simulink model "modelOfSegway"  (R2016a)
settings: Solver=ode45  StartTime=0.0  StopTime=10  RelTol=1e-3
InitFcn:
  | start
  | control
values from neighbouring files (symbols this model uses):
  A = [0 0 1 ... (first row only)    [start.m]
  B = [0 ... (first row only)    [start.m]
  C = eye(3)    [start.m]
  D = 0.07    [params.m]    (also in start.m = zeros(3, 1))
  K = lqr(s1, QQ, RR)    [control.m]    (also in controlEV3.m = lqrd(s1.A,s1.B, QQ, RR, Ts); control_A.m = QQ*Inv(Y)*; control_P.m = (inv(AA)*BB)')
  K_PWM = 8.087    [params.m]
  Psi0 = 0.15    [params.m]
  R = 0.0275    [params.m]
  W = 0.08    [params.m]
libraries: simulink_extras x2
settings Model: Creator=Влад  LastModifiedBy=Влад
settings SolverCC: ZeroCrossAlgorithm=Adaptive

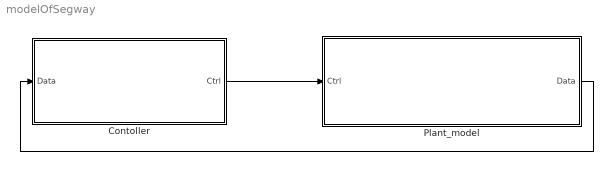
== system modelOfSegway ==
  Contoller : Subsystem
  Plant_model : Subsystem
  wires:
  Contoller/1(Ctrl) -> Plant_model/1(Ctrl)
  Plant_model/1(Data) -> Contoller/1(Data)

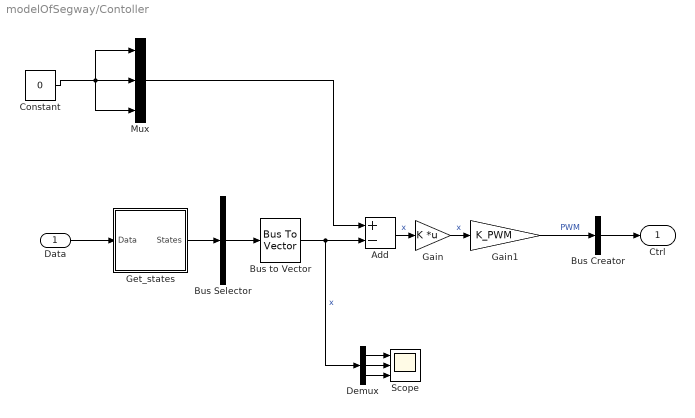
== system modelOfSegway/Contoller ==
  Data : Inport
  Add : Sum  Inputs=+-
  Bus Creator : BusCreator  Inputs=1  OutDataTypeStr=Bus: Ctrl
  Bus Selector : BusSelector  OutputSignals=psi,theta_dot,psi_dot  OutputAsBus=on
  Bus to Vector : BusToVector
  Constant : Constant  Value=0
  Demux : Demux  Outputs=3
  Gain : Gain  Gain=K  Multiplication=Matrix(K*u)
  Gain1 : Gain  Gain=K_PWM
  Get_states : Subsystem
  Mux : Mux  Inputs=3
  Scope : Scope  NumInputPorts=3
  Ctrl : Outport
  wires:
  Bus Creator/1 -> Ctrl/1
  Data/1 -> Get_states/1(Data)
  Get_states/1(States) -> Bus Selector/1
  Bus Selector/1 -> Bus to Vector/1
  Bus to Vector/1 -> Demux/1, Add/2  "x"
  Mux/1 -> Add/1
  Gain1/1 -> Bus Creator/1  "PWM"
  Constant/1 -> Mux/1, Mux/3, Mux/2
  Demux/1 -> Scope/1
  Demux/2 -> Scope/2
  Demux/3 -> Scope/3
  Add/1 -> Gain/1  "x"
  Gain/1 -> Gain1/1  "x"

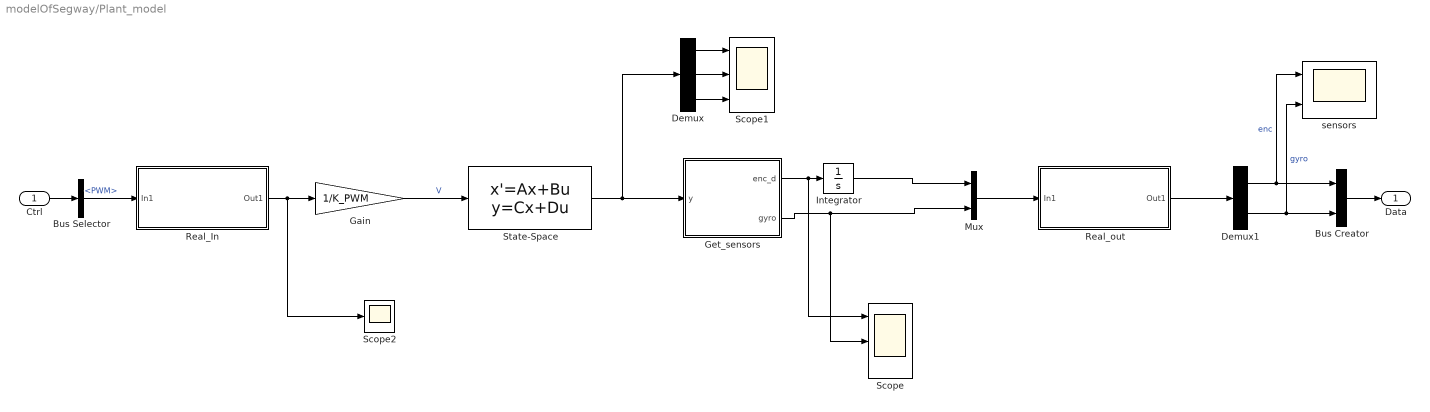
== system modelOfSegway/Plant_model ==
  Ctrl : Inport
  Bus Creator : BusCreator  Inputs=2  OutDataTypeStr=Bus: Data
  Bus Selector : BusSelector  OutputSignals=PWM
  Demux : Demux  Outputs=3
  Demux1 : Demux  Outputs=2
  Gain : Gain  Gain=1/K_PWM
  Get_sensors : MATLAB Function  TreatAsAtomicUnit=on
  Integrator : Integrator
  Mux : Mux  Inputs=2
  Real_In : Subsystem  Variant=on
  Real_out : Subsystem  Variant=on
  Scope : Scope  NumInputPorts=3
  Scope1 : Scope  NumInputPorts=3
  Scope2 : Scope
  State-Space : StateSpace  A=A  B=B  C=C  D=D  X0=[Psi0 0 0]
  "sensors " : Scope  NumInputPorts=2
  Data : Outport
  wires:
  Gain/1 -> State-Space/1  "V"
  Get_sensors/1(enc_d) -> Scope/1, Integrator/1
  Get_sensors/2(gyro) -> Scope/2, Mux/2
  Ctrl/1 -> Bus Selector/1
  Integrator/1 -> Mux/1
  Mux/1 -> Real_out/1(In1)
  Real_out/1(Out1) -> Demux1/1
  Demux1/2 -> "sensors "/2, Bus Creator/2  "gyro"
  Demux1/1 -> "sensors "/1, Bus Creator/1  "enc"
  Bus Creator/1 -> Data/1
  Bus Selector/1 -> Real_In/1(In1)  "<PWM>"
  Real_In/1(Out1) -> Scope2/1, Gain/1
  State-Space/1 -> Demux/1, Get_sensors/1(y)
  Demux/1 -> Scope1/1
  Demux/2 -> Scope1/2
  Demux/3 -> Scope1/3

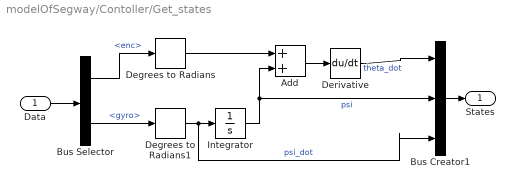
== system modelOfSegway/Contoller/Get_states ==
  Data : Inport
  Add : Sum
  Bus Creator1 : BusCreator  Inputs=3
  Bus Selector : BusSelector  OutputSignals=enc,gyro
  Degrees to Radians : simulink_extras/Transformations/Degrees to Radians
  Degrees to Radians1 : simulink_extras/Transformations/Degrees to Radians
  Derivative : Derivative
  Integrator : Integrator
  States : Outport
  wires:
  Bus Selector/2 -> Degrees to Radians1/1  "<gyro>"
  Data/1 -> Bus Selector/1
  Bus Selector/1 -> Degrees to Radians/1  "<enc>"
  Degrees to Radians/1 -> Add/1
  Integrator/1 -> Bus Creator1/2, Add/2  "psi"
  Degrees to Radians1/1 -> Bus Creator1/3, Integrator/1  "psi_dot"
  Bus Creator1/1 -> States/1
  Derivative/1 -> Bus Creator1/1  "theta_dot"
  Add/1 -> Derivative/1

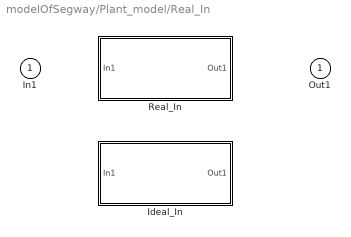
== system modelOfSegway/Plant_model/Real_In ==
  In1 : Inport
  Ideal_In : Subsystem  VariantControl=(default)
  Real_In : Subsystem  VariantControl=real_model == 1
  Out1 : Outport

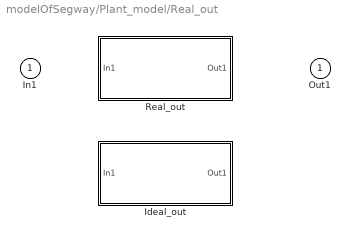
== system modelOfSegway/Plant_model/Real_out ==
  In1 : Inport
  Ideal_out : Subsystem  VariantControl=(default)
  Real_out : Subsystem  VariantControl=real_model == 1
  Out1 : Outport

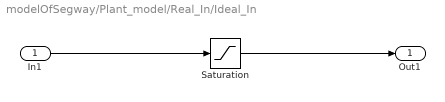
== system modelOfSegway/Plant_model/Real_In/Ideal_In ==
  In1 : Inport
  Saturation : Saturate  UpperLimit=100  LowerLimit=-100
  Out1 : Outport
  wires:
  In1/1 -> Saturation/1
  Saturation/1 -> Out1/1

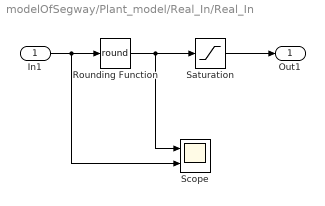
== system modelOfSegway/Plant_model/Real_In/Real_In ==
  In1 : Inport
  Rounding Function : Rounding  Operator=round
  Saturation : Saturate  UpperLimit=100  LowerLimit=-100
      settings: LockScale=on
  Scope : Scope  NumInputPorts=2
  Out1 : Outport
  wires:
  In1/1 -> Scope/2, Rounding Function/1
  Saturation/1 -> Out1/1
  Rounding Function/1 -> Scope/1, Saturation/1

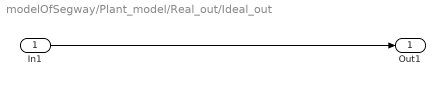
== system modelOfSegway/Plant_model/Real_out/Ideal_out ==
  In1 : Inport
  Out1 : Outport
  wires:
  In1/1 -> Out1/1

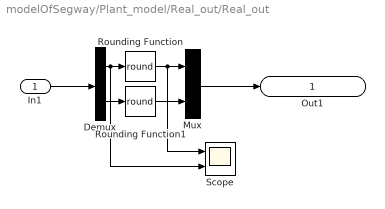
== system modelOfSegway/Plant_model/Real_out/Real_out ==
  In1 : Inport
  Demux : Demux  Outputs=2
  Mux : Mux  Inputs=2
  Rounding Function : Rounding  Operator=round
  Rounding Function1 : Rounding  Operator=round
  Scope : Scope  NumInputPorts=2
  Out1 : Outport
  wires:
  In1/1 -> Demux/1
  Demux/1 -> Scope/2, Rounding Function/1
  Demux/2 -> Rounding Function1/1
  Rounding Function1/1 -> Mux/2
  Rounding Function/1 -> Scope/1, Mux/1
  Mux/1 -> Out1/1

== matlab function modelOfSegway/Plant_model/Get_sensors ==
  data: y input; enc_d output; gyro output; W parameter; R parameter
function [enc_d, gyro] = sensors(y, W, R)
%#codegen 'psi', 'theta_dot', 'psi_dot'
enc_d = rad2deg(y(2));
gyro = rad2deg(y(3));
